simulink model "VSCHVDCunitblackstart"  (R2025b)
settings: Solver=VariableStepAuto  StartTime=0  StopTime=25  FixedStep=5e-5  RelTol=1e-3
PreLoadFcn:
  | HVDCParameters;
  | BlackStartMMCParameters;
undefined symbols (not defined in the file): DiscIntNeverNeededParam, FRated, frt, gGFM, grid, Lbase, Lr, Lt, lvrt, mGFM, mpptOmega, mpptWindSpeed, Nm, pmsm, PRated, Rc, rpir, Rr, Rt, time, Tpir, Ts, Vbase, Vdcs0, VRated, Vt2, windController, windTurbine, Zbase
libraries: fl_lib x47, ee_lib x41, nesl_utility x33, eeGeneralControl x13, eeTransforms x12, slpidlib x8, eeSinusoidalMeasurementV2 x4, simulink x2, eeSinusoidalMeasurement x1, eeStairGenerator x1
(part 4 of 5)

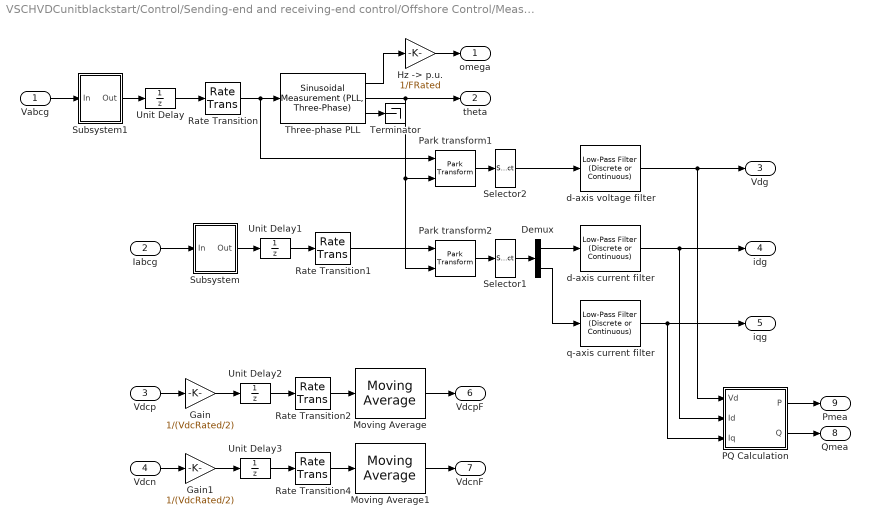
== system VSCHVDCunitblackstart/Control/Sending-end and receiving-end control/Offshore Control/Measurements ==
  Vabcg : Inport
  Iabcg : Inport  Port=2
  Vdcp : Inport  Port=3
  Vdcn : Inport  Port=4
  Demux : Demux  Outputs=2
  Gain : Gain  Gain=1/(VdcRated/2)
  Gain1 : Gain  Gain=1/(VdcRated/2)
  "Hz -> p.u." : Gain  Gain=1/FRated
  Moving Average : eeGeneralControl/Moving Average  VariantControl=Variant1  LabelModeActiveChoice=Discrete  f=FRated  x0=Vdcr0/2/(VdcRated/2)  BufferSize=8192  Ts=Tsc
  Moving Average1 : eeGeneralControl/Moving Average  VariantControl=Variant1  LabelModeActiveChoice=Discrete  f=FRated  x0=Vdcr0/2/(VdcRated/2)  BufferSize=8192  Ts=Tsc
  PQ Calculation : Subsystem
  Park transform1 : eeTransforms/Park Transform  AxisAlignment=Q-axis  PowerInvariant=off
  Park transform2 : eeTransforms/Park Transform  AxisAlignment=Q-axis  PowerInvariant=off
  Rate Transition : RateTransition  InitialCondition=Vabcgr0  OutPortSampleTime=Tsc
  Rate Transition1 : RateTransition  InitialCondition=Iabcgr0  OutPortSampleTime=Tsc
  Rate Transition2 : RateTransition  InitialCondition=Vdcr0/2/(VdcRated/2)  OutPortSampleTime=Tsc
  Rate Transition4 : RateTransition  InitialCondition=Vdcr0/2/(VdcRated/2)  OutPortSampleTime=Tsc
  Selector1 : Selector  InputPortWidth=3  IndexOptions=Index vector (dialog)  Indices=[1 2]  OutputSizes=1
  Selector2 : Selector  InputPortWidth=3  IndexOptions=Index vector (dialog)  Indices=[1]  OutputSizes=1
  Subsystem : Subsystem
  Subsystem1 : Subsystem
  Terminator : Terminator
  Three-phase PLL : eeSinusoidalMeasurement/Sinusoidal Measurement (PLL, Three-Phase)  Kp_LF=45  Ki_LF=1250  F0=FRated  Theta0=Vphaser0  Ts=Tsc
  Unit Delay : UnitDelay  InitialCondition=Vabcgr0  SampleTime=Ts  HasFrameUpgradeWarning=on
  Unit Delay1 : UnitDelay  InitialCondition=Iabcgr0  SampleTime=Ts  HasFrameUpgradeWarning=on
  Unit Delay2 : UnitDelay  InitialCondition=Vdcr0/2/(VdcRated/2)  SampleTime=Ts  HasFrameUpgradeWarning=on
  Unit Delay3 : UnitDelay  InitialCondition=Vdcr0/2/(VdcRated/2)  SampleTime=Ts  HasFrameUpgradeWarning=on
  d-axis current filter : eeGeneralControl/Low-Pass Filter (Discrete or Continuous)  K=1  T=5e-3  B=inf  A=-inf  init_option=Specify as parameter  x0=0  Ts=Tsc
  d-axis voltage filter : eeGeneralControl/Low-Pass Filter (Discrete or Continuous)  K=1  T=5e-3  B=inf  A=-inf  init_option=Specify as parameter  x0=0  Ts=Tsc
  q-axis current filter : eeGeneralControl/Low-Pass Filter (Discrete or Continuous)  K=1  T=5e-3  B=inf  A=-inf  init_option=Specify as parameter  x0=0  Ts=Tsc
  omega : Outport  VectorParamsAs1DForOutWhenUnconnected=off
  theta : Outport  Port=2  VectorParamsAs1DForOutWhenUnconnected=off
  Vdg : Outport  Port=3  VectorParamsAs1DForOutWhenUnconnected=off
  idg : Outport  Port=4  VectorParamsAs1DForOutWhenUnconnected=off
  iqg : Outport  Port=5  VectorParamsAs1DForOutWhenUnconnected=off
  VdcpF : Outport  Port=6  VectorParamsAs1DForOutWhenUnconnected=off
  VdcnF : Outport  Port=7  VectorParamsAs1DForOutWhenUnconnected=off
  Qmea : Outport  Port=8  VectorParamsAs1DForOutWhenUnconnected=off
  Pmea : Outport  Port=9  VectorParamsAs1DForOutWhenUnconnected=off
  wires:
  Moving Average1/1 -> VdcnF/1
  Vdcn/1 -> Gain1/1
  Rate Transition4/1 -> Moving Average1/1
  Gain1/1 -> Unit Delay3/1
  PQ Calculation/2(Q) -> Qmea/1
  PQ Calculation/1(P) -> Pmea/1
  Selector2/1 -> d-axis voltage filter/1
  d-axis current filter/1 -> idg/1, PQ Calculation/2(Id)
  Rate Transition1/1 -> Park transform2/1
  Rate Transition/1 -> Three-phase PLL/1, Park transform1/1
  d-axis voltage filter/1 -> PQ Calculation/1(Vd), Vdg/1
  Park transform2/1 -> Selector1/1
  Demux/1 -> d-axis current filter/1
  Gain/1 -> Unit Delay2/1
  Vdcp/1 -> Gain/1
  Demux/2 -> q-axis current filter/1
  Three-phase PLL/1 -> "Hz -> p.u."/1
  Park transform1/1 -> Selector2/1
  Three-phase PLL/2 -> Park transform1/2, Park transform2/2, theta/1
  Selector1/1 -> Demux/1
  Three-phase PLL/3 -> Terminator/1
  Moving Average/1 -> VdcpF/1
  "Hz -> p.u."/1 -> omega/1
  Iabcg/1 -> Subsystem/1(In)
  Vabcg/1 -> Subsystem1/1(In)
  Rate Transition2/1 -> Moving Average/1
  q-axis current filter/1 -> iqg/1, PQ Calculation/3(Iq)
  Unit Delay2/1 -> Rate Transition2/1
  Unit Delay3/1 -> Rate Transition4/1
  Unit Delay/1 -> Rate Transition/1
  Subsystem/1(Out) -> Unit Delay1/1
  Unit Delay1/1 -> Rate Transition1/1
  Subsystem1/1(Out) -> Unit Delay/1

== system VSCHVDCunitblackstart/Control/Sending-end and receiving-end control/Onshore Control/Control ==
  Vdref : Inport
  Vqref : Inport  Port=2
  Vdcp : Inport  Port=3
  Vdcn : Inport  Port=4
  Vdmea : Inport  Port=5
  Vqmea : Inport  Port=6
  theta : Inport  Port=7
  Active and reactive power control : Subsystem
  Add3 : Sum
  Constant : Constant  Value=0  SampleTime=Tsc
  Divide : Product  Inputs=*/
  Gain : Gain  Gain=2
  Gain5 : Gain  Gain=0.5*VdcRated/Vbase
  Inverse Park Transform : eeTransforms/Inverse Park Transform  AxisAlignment=Q-axis  PowerInvariant=off
  Mux1 : Mux  Inputs=3
  PWM generator : Subsystem
  S : Outport
  wires:
  Vdmea/1 -> Active and reactive power control/2(Vdmea)
  Vqmea/1 -> Active and reactive power control/4(Vqmea)
  PWM generator/1(S) -> S/1
  Vdref/1 -> Active and reactive power control/1(Vd)
  Vqref/1 -> Active and reactive power control/3(Vqref)
  Vdcn/1 -> Add3/2
  Vdcp/1 -> Add3/1
  Inverse Park Transform/1 -> Divide/1
  Gain5/1 -> Divide/2
  Add3/1 -> Gain5/1
  Divide/1 -> Gain/1
  Gain/1 -> PWM generator/1(Vref)
  Mux1/1 -> Inverse Park Transform/1
  theta/1 -> Inverse Park Transform/2
  Active and reactive power control/1(idRef) -> Mux1/1
  Constant/1 -> Mux1/3
  Active and reactive power control/2(iqRef) -> Mux1/2

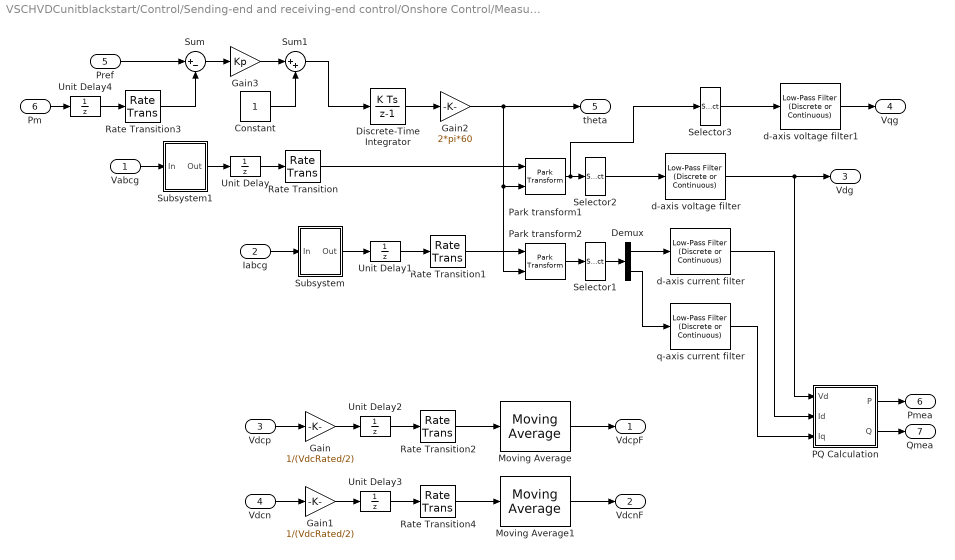
== system VSCHVDCunitblackstart/Control/Sending-end and receiving-end control/Onshore Control/Measurements ==
  Vabcg : Inport
  Iabcg : Inport  Port=2
  Vdcp : Inport  Port=3
  Vdcn : Inport  Port=4
  Pref : Inport  Port=5
  Pm : Inport  Port=6
  Constant : Constant
  Demux : Demux  Outputs=2
  Discrete-Time Integrator : DiscreteIntegrator  InitialCondition=1  SampleTime=-1  ICPrevOutput=DiscIntNeverNeededParam  ICPrevScaledInput=DiscIntNeverNeededParam
  Gain : Gain  Gain=1/(VdcRated/2)
  Gain1 : Gain  Gain=1/(VdcRated/2)
  Gain2 : Gain  Gain=2*pi*60
  Gain3 : Gain  Gain=Kp
  Moving Average : eeGeneralControl/Moving Average  VariantControl=Variant1  LabelModeActiveChoice=Discrete  f=FRated  x0=Vdcs0/2/(VdcRated/2)  BufferSize=8192  Ts=Tsc
  Moving Average1 : eeGeneralControl/Moving Average  VariantControl=Variant1  LabelModeActiveChoice=Discrete  f=FRated  x0=Vdcs0/2/(VdcRated/2)  BufferSize=8192  Ts=Tsc
  PQ Calculation : Subsystem
  Park transform1 : eeTransforms/Park Transform  AxisAlignment=Q-axis  PowerInvariant=off
  Park transform2 : eeTransforms/Park Transform  AxisAlignment=Q-axis  PowerInvariant=off
  Rate Transition : RateTransition  InitialCondition=Vabcgs0  OutPortSampleTime=Tsc
  Rate Transition1 : RateTransition  InitialCondition=Iabcgs0  OutPortSampleTime=Tsc
  Rate Transition2 : RateTransition  InitialCondition=Vdcs0/2/(VdcRated/2)  OutPortSampleTime=Tsc
  Rate Transition3 : RateTransition  InitialCondition=Vabcgs0  OutPortSampleTime=Tsc
  Rate Transition4 : RateTransition  InitialCondition=Vdcs0/2/(VdcRated/2)  OutPortSampleTime=Tsc
  Selector1 : Selector  InputPortWidth=3  IndexOptions=Index vector (dialog)  Indices=[1 2]  OutputSizes=1
  Selector2 : Selector  InputPortWidth=3  IndexOptions=Index vector (dialog)  Indices=[1]  OutputSizes=1
  Selector3 : Selector  InputPortWidth=3  IndexOptions=Index vector (dialog)  Indices=[2]  OutputSizes=1
  Subsystem : Subsystem
  Subsystem1 : Subsystem
  Sum : Sum  Inputs=|+-
  Sum1 : Sum  Inputs=|++
  Unit Delay : UnitDelay  InitialCondition=Vabcgs0  SampleTime=Ts  HasFrameUpgradeWarning=on
  Unit Delay1 : UnitDelay  InitialCondition=Iabcgs0  SampleTime=Ts  HasFrameUpgradeWarning=on
  Unit Delay2 : UnitDelay  InitialCondition=Vdcs0/2/(VdcRated/2)  SampleTime=Ts  HasFrameUpgradeWarning=on
  Unit Delay3 : UnitDelay  InitialCondition=Vdcs0/2/(VdcRated/2)  SampleTime=Ts  HasFrameUpgradeWarning=on
  Unit Delay4 : UnitDelay  InitialCondition=Vabcgs0  SampleTime=Ts  HasFrameUpgradeWarning=on
  d-axis current filter : eeGeneralControl/Low-Pass Filter (Discrete or Continuous)  K=1  T=5e-3  B=inf  A=-inf  init_option=Specify as parameter  x0=0  Ts=Tsc
  d-axis voltage filter : eeGeneralControl/Low-Pass Filter (Discrete or Continuous)  K=1  T=5e-3  B=inf  A=-inf  init_option=Specify as parameter  x0=0  Ts=Tsc
  d-axis voltage filter1 : eeGeneralControl/Low-Pass Filter (Discrete or Continuous)  K=1  T=5e-3  B=inf  A=-inf  init_option=Specify as parameter  x0=0  Ts=Tsc
  q-axis current filter : eeGeneralControl/Low-Pass Filter (Discrete or Continuous)  K=1  T=5e-3  B=inf  A=-inf  init_option=Specify as parameter  x0=0  Ts=Tsc
  VdcpF : Outport  VectorParamsAs1DForOutWhenUnconnected=off
  VdcnF : Outport  Port=2  VectorParamsAs1DForOutWhenUnconnected=off
  Vdg : Outport  Port=3  VectorParamsAs1DForOutWhenUnconnected=off
  Vqg : Outport  Port=4  VectorParamsAs1DForOutWhenUnconnected=off
  theta : Outport  Port=5  VectorParamsAs1DForOutWhenUnconnected=off
  Pmea : Outport  Port=6  VectorParamsAs1DForOutWhenUnconnected=off
  Qmea : Outport  Port=7  VectorParamsAs1DForOutWhenUnconnected=off
  wires:
  Rate Transition2/1 -> Moving Average/1
  Iabcg/1 -> Subsystem/1(In)
  Selector1/1 -> Demux/1
  Park transform1/1 -> Selector3/1, Selector2/1
  Demux/2 -> q-axis current filter/1
  Vdcp/1 -> Gain/1
  Demux/1 -> d-axis current filter/1
  Park transform2/1 -> Selector1/1
  d-axis voltage filter/1 -> Vdg/1, PQ Calculation/1(Vd)
  Rate Transition/1 -> Park transform1/1
  Rate Transition1/1 -> Park transform2/1
  Selector2/1 -> d-axis voltage filter/1
  PQ Calculation/1(P) -> Pmea/1
  PQ Calculation/2(Q) -> Qmea/1
  Rate Transition4/1 -> Moving Average1/1
  Vdcn/1 -> Gain1/1
  Discrete-Time Integrator/1 -> Gain2/1
  Unit Delay/1 -> Rate Transition/1
  Unit Delay2/1 -> Rate Transition2/1
  Unit Delay3/1 -> Rate Transition4/1
  Gain/1 -> Unit Delay2/1
  Gain1/1 -> Unit Delay3/1
  Vabcg/1 -> Subsystem1/1(In)
  Subsystem/1(Out) -> Unit Delay1/1
  d-axis current filter/1 -> PQ Calculation/2(Id)
  q-axis current filter/1 -> PQ Calculation/3(Iq)
  Moving Average/1 -> VdcpF/1
  Moving Average1/1 -> VdcnF/1
  Unit Delay1/1 -> Rate Transition1/1
  Subsystem1/1(Out) -> Unit Delay/1
  Gain2/1 -> Park transform2/2, Park transform1/2, theta/1
  Pref/1 -> Sum/1
  Pm/1 -> Unit Delay4/1
  Sum/1 -> Gain3/1
  Gain3/1 -> Sum1/1
  Sum1/1 -> Discrete-Time Integrator/1
  Constant/1 -> Sum1/2
  Rate Transition3/1 -> Sum/2
  Unit Delay4/1 -> Rate Transition3/1
  Selector3/1 -> d-axis voltage filter1/1
  d-axis voltage filter1/1 -> Vqg/1

== system VSCHVDCunitblackstart/Wind Farm/Wind Farm/CB1/Subsystem1 ==
  input0 : Inport
  Gain : Gain  Gain=1e9
  Phase Splitter : ee_lib/Connectors & References/Phase Splitter
  Phase Splitter1 : ee_lib/Connectors & References/Phase Splitter
  Simulink-PS Converter : nesl_utility/Simulink-PS Converter  PhysicalDomain=network_engine_domain  SubClassName=ps_input  LeftPortType=input  RightPortType=output  PseudoPeriodic=off  Frequencies=[]  NoiseDistribution=none  NoiseParameters=[]  Unit=1  AffineConversion=off  FilteringAndDerivatives=provide  SimscapeFilterOrder=1  InputFilterTimeConstant=0.001  UdotUserProvided=0
  Variable Resistor : fl_lib/Electrical/Electrical Elements/Variable Resistor  Rmin=1e-4 Ohm  thermalEnable=false  thermal_mass=1 J/K  i_specify=off  i_priority=None  i=0 A  i_nominal_specify=off  i_nominal_value=1  i_nominal_unit=A  v_specify=off  v_priority=None  v=0 V  v_nominal_specify=off  v_nominal_value=1  v_nominal_unit=V  T_specify=off  T_priority=None  T=300 K  T_nominal_specify=off  T_nominal_value=1  T_nominal_unit=K
  Variable Resistor1 : fl_lib/Electrical/Electrical Elements/Variable Resistor  Rmin=1e-4 Ohm  thermalEnable=false  thermal_mass=1 J/K  i_specify=off  i_priority=None  i=0 A  i_nominal_specify=off  i_nominal_value=1  i_nominal_unit=A  v_specify=off  v_priority=None  v=0 V  v_nominal_specify=off  v_nominal_value=1  v_nominal_unit=V  T_specify=off  T_priority=None  T=300 K  T_nominal_specify=off  T_nominal_value=1  T_nominal_unit=K
  Variable Resistor2 : fl_lib/Electrical/Electrical Elements/Variable Resistor  Rmin=1e-4 Ohm  thermalEnable=false  thermal_mass=1 J/K  i_specify=off  i_priority=None  i=0 A  i_nominal_specify=off  i_nominal_value=1  i_nominal_unit=A  v_specify=off  v_priority=None  v=0 V  v_nominal_specify=off  v_nominal_value=1  v_nominal_unit=V  T_specify=off  T_priority=None  T=300 K  T_nominal_specify=off  T_nominal_value=1  T_nominal_unit=K
  Conn1 : PMIOPort  Side=Left
  Conn2 : PMIOPort  Port=2  Side=Right
  wires:
  input0/1 -> Gain/1
  Gain/1 -> Simulink-PS Converter/1
  connections:
  Simulink-PS Converter/RConn1 -- Variable Resistor2/LConn1 -- Variable Resistor1/LConn1 -- Variable Resistor/LConn1
  Phase Splitter/LConn1 -- Conn2/RConn1
  Phase Splitter/RConn1 -- Variable Resistor/LConn2
  Phase Splitter/RConn2 -- Variable Resistor1/LConn2
  Phase Splitter/RConn3 -- Variable Resistor2/LConn2
  Phase Splitter1/LConn1 -- Conn1/RConn1
  Variable Resistor/RConn1 -- Phase Splitter1/RConn1
  Phase Splitter1/RConn2 -- Variable Resistor1/RConn1
  Variable Resistor2/RConn1 -- Phase Splitter1/RConn3

== system VSCHVDCunitblackstart/Wind Farm/Wind Farm/PLL & Measurements/Measurement1 ==
  u : Inport
  Ig : Outport
  wires:
  u/1 -> Ig/1

== system VSCHVDCunitblackstart/Wind Farm/Wind Farm/PLL & Measurements/Measurement2 ==
  u : Inport
  Vg : Outport
  wires:
  u/1 -> Vg/1

== system VSCHVDCunitblackstart/Wind Farm/Wind Farm/PLL & Measurements/PLL ==
  abc : Inport
  Ig : Inport  Port=2
  Demux : Demux  Outputs=3
  Demux1 : Demux  Outputs=3
  Park Transform : eeTransforms/Park Transform  AxisAlignment=Q-axis  PowerInvariant=off
  Park Transform1 : eeTransforms/Park Transform  AxisAlignment=Q-axis  PowerInvariant=off
  "Sinusoidal Measurement (PLL, Three-Phase)1" : eeSinusoidalMeasurementV2/Sinusoidal Measurement (PLL, Three-Phase)  InputFilter=on  InputNormalization=off  Kp_LF=pll.kp  Ki_LF=pll.ki  F0=grid.frequency  Theta0=0  Ts=Ts
      settings: LibrarySourceBlock=|
      | ee_sl_lib/Measurements/Sinusoidal Measurement
      | (PLL, Three-Phase)
  Terminator : Terminator
  Terminator1 : Terminator
  abc1 : InportShadow
  mag : Outport
  freq : Outport  Port=2
  angle : Outport  Port=3
  Vd : Outport  Port=4
  Vq : Outport  Port=5
  Id : Outport  Port=6
  Iq : Outport  Port=7
  wires:
  Demux/3 -> Terminator/1
  Park Transform/1 -> Demux/1
  Demux/1 -> Vd/1
  Demux/2 -> Vq/1
  "Sinusoidal Measurement (PLL, Three-Phase)1"/3 -> mag/1
  "Sinusoidal Measurement (PLL, Three-Phase)1"/2 -> angle/1, Park Transform/2, Park Transform1/2
  Ig/1 -> Park Transform1/1
  Demux1/2 -> Iq/1
  Park Transform1/1 -> Demux1/1
  Demux1/1 -> Id/1
  Demux1/3 -> Terminator1/1
  abc1/1 -> Park Transform/1
  abc/1 -> "Sinusoidal Measurement (PLL, Three-Phase)1"/1
  "Sinusoidal Measurement (PLL, Three-Phase)1"/1 -> freq/1

== system VSCHVDCunitblackstart/Wind Farm/Wind Farm/Voltage VAR Control & LVRT, FRT/Frequency RideThrough ==
  f : Inport
  Avoid Operation : Subsystem
  Discrete-Time Integrator1 : DiscreteIntegrator  ExternalReset=either  SampleTime=Ts  ICPrevOutput=DiscIntNeverNeededParam  ICPrevScaledInput=DiscIntNeverNeededParam
  Duration of f<fth : Lookup_n-D  NumberOfTableDimensions=1  BreakpointsForDimension1=(1+[-0.021,-0.02,0.02,0.021])*grid.frequency  Table=[1,0,0,1]  InterpMethod=Flat  InternalRulePriority=Speed  RndMeth=Simplest
  Frequency vs Trip time : Lookup_n-D  NumberOfTableDimensions=1  BreakpointsForDimension1=frt.frequency  Table=frt.time  InterpMethod=Flat  InternalRulePriority=Speed  RndMeth=Simplest
  GreaterThan : RelationalOperator  Operator=>  OutDataTypeStr=boolean  RndMeth=Simplest  InputSameDT=off
  Trip  Signal : Outport
  wires:
  Discrete-Time Integrator1/1 -> GreaterThan/1
  Frequency vs Trip time/1 -> GreaterThan/2
  GreaterThan/1 -> Trip  Signal/1
  Duration of f<fth/1 -> Discrete-Time Integrator1/2, Discrete-Time Integrator1/1
  Avoid Operation/1(f) -> Duration of f<fth/1, Frequency vs Trip time/1
  f/1 -> Avoid Operation/1(f_in)

== system VSCHVDCunitblackstart/Wind Farm/Wind Farm/Voltage VAR Control & LVRT, FRT/LVRT Characterstics ==
  Vmag : Inport
  Discrete-Time Integrator1 : DiscreteIntegrator  ExternalReset=either  SampleTime=Ts  ICPrevOutput=DiscIntNeverNeededParam  ICPrevScaledInput=DiscIntNeverNeededParam
  Duration of Vmag<Vth : Lookup_n-D  NumberOfTableDimensions=1  BreakpointsForDimension1=[0,.9,0.91,1.2]  Table=[1,1,0,0]  InterpMethod=Flat  InternalRulePriority=Speed  RndMeth=Simplest
  Gain1 : Gain  Gain=-1
  GreaterThan : RelationalOperator  Operator=>  OutDataTypeStr=boolean  RndMeth=Simplest  InputSameDT=off
  Saturation2 : Saturate  UpperLimit=1/8  LowerLimit=-1
  Vmag vs Trip time : Lookup_n-D  NumberOfTableDimensions=1  BreakpointsForDimension1=lvrt.voltage  Table=lvrt.time  InterpMethod=Flat  InternalRulePriority=Speed  RndMeth=Simplest
  Vmag vs iq : Lookup_n-D  NumberOfTableDimensions=1  BreakpointsForDimension1=lvrt.voltageiq  Table=lvrt.iq  InternalRulePriority=Speed  RndMeth=Simplest
  Trip Signal : Outport
  iq : Outport  Port=2
  wires:
  Duration of Vmag<Vth/1 -> Discrete-Time Integrator1/2, Discrete-Time Integrator1/1
  GreaterThan/1 -> Trip Signal/1
  Discrete-Time Integrator1/1 -> GreaterThan/1
  Vmag vs Trip time/1 -> GreaterThan/2
  Vmag vs iq/1 -> Saturation2/1
  Gain1/1 -> iq/1
  Saturation2/1 -> Gain1/1
  Vmag/1 -> Vmag vs iq/1, Vmag vs Trip time/1, Duration of Vmag<Vth/1

== system VSCHVDCunitblackstart/Wind Farm/Wind Farm/Voltage VAR Control & LVRT, FRT/Voltage Control ==
  In1 : Inport
  In2 : Inport  Port=2
  Constant2 : Constant  Value=0
  Gain : Gain  Gain=windController.mv
  Sum2 : Sum  Inputs=|+-
  Switch1 : Switch  Threshold=.9  SaturateOnIntegerOverflow=off  InputSameDT=off
  Out1 : Outport
  wires:
  Gain/1 -> Out1/1
  Sum2/1 -> Switch1/1
  Switch1/1 -> Gain/1
  In1/1 -> Sum2/2, Switch1/2
  Constant2/1 -> Switch1/3
  In2/1 -> Sum2/1

== system VSCHVDCunitblackstart/Wind Farm/Wind Farm1/CB1/Subsystem1 ==
  input0 : Inport
  Gain : Gain  Gain=1e9
  Phase Splitter : ee_lib/Connectors & References/Phase Splitter
  Phase Splitter1 : ee_lib/Connectors & References/Phase Splitter
  Simulink-PS Converter : nesl_utility/Simulink-PS Converter  PhysicalDomain=network_engine_domain  SubClassName=ps_input  LeftPortType=input  RightPortType=output  PseudoPeriodic=off  Frequencies=[]  NoiseDistribution=none  NoiseParameters=[]  Unit=1  AffineConversion=off  FilteringAndDerivatives=provide  SimscapeFilterOrder=1  InputFilterTimeConstant=0.001  UdotUserProvided=0
  Variable Resistor : fl_lib/Electrical/Electrical Elements/Variable Resistor  Rmin=1e-4 Ohm  thermalEnable=false  thermal_mass=1 J/K  i_specify=off  i_priority=None  i=0 A  i_nominal_specify=off  i_nominal_value=1  i_nominal_unit=A  v_specify=off  v_priority=None  v=0 V  v_nominal_specify=off  v_nominal_value=1  v_nominal_unit=V  T_specify=off  T_priority=None  T=300 K  T_nominal_specify=off  T_nominal_value=1  T_nominal_unit=K
  Variable Resistor1 : fl_lib/Electrical/Electrical Elements/Variable Resistor  Rmin=1e-4 Ohm  thermalEnable=false  thermal_mass=1 J/K  i_specify=off  i_priority=None  i=0 A  i_nominal_specify=off  i_nominal_value=1  i_nominal_unit=A  v_specify=off  v_priority=None  v=0 V  v_nominal_specify=off  v_nominal_value=1  v_nominal_unit=V  T_specify=off  T_priority=None  T=300 K  T_nominal_specify=off  T_nominal_value=1  T_nominal_unit=K
  Variable Resistor2 : fl_lib/Electrical/Electrical Elements/Variable Resistor  Rmin=1e-4 Ohm  thermalEnable=false  thermal_mass=1 J/K  i_specify=off  i_priority=None  i=0 A  i_nominal_specify=off  i_nominal_value=1  i_nominal_unit=A  v_specify=off  v_priority=None  v=0 V  v_nominal_specify=off  v_nominal_value=1  v_nominal_unit=V  T_specify=off  T_priority=None  T=300 K  T_nominal_specify=off  T_nominal_value=1  T_nominal_unit=K
  Conn1 : PMIOPort  Side=Left
  Conn2 : PMIOPort  Port=2  Side=Right
  wires:
  input0/1 -> Gain/1
  Gain/1 -> Simulink-PS Converter/1
  connections:
  Simulink-PS Converter/RConn1 -- Variable Resistor2/LConn1 -- Variable Resistor1/LConn1 -- Variable Resistor/LConn1
  Phase Splitter/LConn1 -- Conn2/RConn1
  Phase Splitter/RConn1 -- Variable Resistor/LConn2
  Phase Splitter/RConn2 -- Variable Resistor1/LConn2
  Phase Splitter/RConn3 -- Variable Resistor2/LConn2
  Phase Splitter1/LConn1 -- Conn1/RConn1
  Variable Resistor/RConn1 -- Phase Splitter1/RConn1
  Phase Splitter1/RConn2 -- Variable Resistor1/RConn1
  Variable Resistor2/RConn1 -- Phase Splitter1/RConn3

== system VSCHVDCunitblackstart/Wind Farm/Wind Farm1/PLL & Measurements/Measurement1 ==
  u : Inport
  Ig : Outport
  wires:
  u/1 -> Ig/1

== system VSCHVDCunitblackstart/Wind Farm/Wind Farm1/PLL & Measurements/Measurement2 ==
  u : Inport
  Vg : Outport
  wires:
  u/1 -> Vg/1

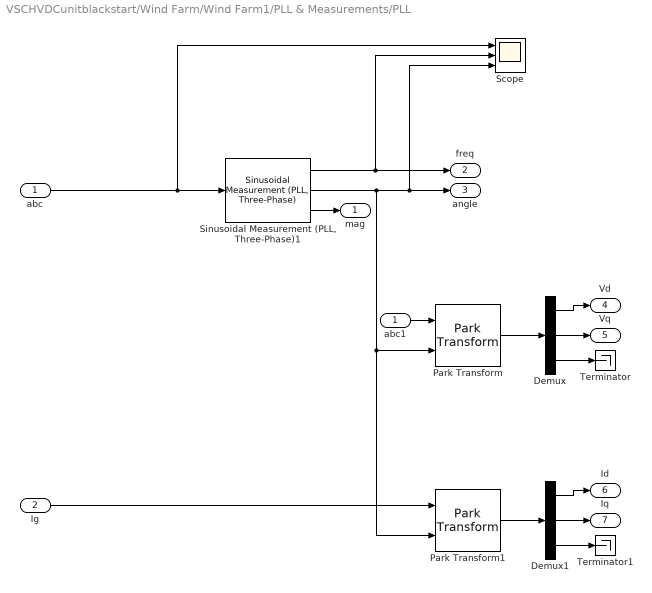
== system VSCHVDCunitblackstart/Wind Farm/Wind Farm1/PLL & Measurements/PLL ==
  abc : Inport
  Ig : Inport  Port=2
  Demux : Demux  Outputs=3
  Demux1 : Demux  Outputs=3
  Park Transform : eeTransforms/Park Transform  AxisAlignment=Q-axis  PowerInvariant=off
  Park Transform1 : eeTransforms/Park Transform  AxisAlignment=Q-axis  PowerInvariant=off
  Scope : Scope  NumInputPorts=3
      settings: ActiveDisplayYMinimum=-1.5640635972149539  ActiveDisplayYMaximum=1.5640663714492395  DataLoggingVariableName=ScopeData5
  "Sinusoidal Measurement (PLL, Three-Phase)1" : eeSinusoidalMeasurementV2/Sinusoidal Measurement (PLL, Three-Phase)  InputFilter=on  InputNormalization=off  Kp_LF=pll.kp  Ki_LF=pll.ki  F0=grid.frequency  Theta0=0  Ts=Ts
      settings: LibrarySourceBlock=|
      | ee_sl_lib/Measurements/Sinusoidal Measurement
      | (PLL, Three-Phase)
  Terminator : Terminator
  Terminator1 : Terminator
  abc1 : InportShadow
  mag : Outport
  freq : Outport  Port=2
  angle : Outport  Port=3
  Vd : Outport  Port=4
  Vq : Outport  Port=5
  Id : Outport  Port=6
  Iq : Outport  Port=7
  wires:
  Demux/3 -> Terminator/1
  Park Transform/1 -> Demux/1
  Demux/1 -> Vd/1
  Demux/2 -> Vq/1
  "Sinusoidal Measurement (PLL, Three-Phase)1"/3 -> mag/1
  "Sinusoidal Measurement (PLL, Three-Phase)1"/2 -> Scope/3, angle/1, Park Transform/2, Park Transform1/2
  Ig/1 -> Park Transform1/1
  Demux1/2 -> Iq/1
  Park Transform1/1 -> Demux1/1
  Demux1/1 -> Id/1
  Demux1/3 -> Terminator1/1
  abc1/1 -> Park Transform/1
  abc/1 -> Scope/1, "Sinusoidal Measurement (PLL, Three-Phase)1"/1
  "Sinusoidal Measurement (PLL, Three-Phase)1"/1 -> Scope/2, freq/1

== system VSCHVDCunitblackstart/Wind Farm/Wind Farm1/Voltage VAR Control & LVRT, FRT/Frequency RideThrough ==
  f : Inport
  Avoid Operation : Subsystem
  Discrete-Time Integrator1 : DiscreteIntegrator  ExternalReset=either  SampleTime=Ts  ICPrevOutput=DiscIntNeverNeededParam  ICPrevScaledInput=DiscIntNeverNeededParam
  Duration of f<fth : Lookup_n-D  NumberOfTableDimensions=1  BreakpointsForDimension1=(1+[-0.021,-0.02,0.02,0.021])*grid.frequency  Table=[1,0,0,1]  InterpMethod=Flat  InternalRulePriority=Speed  RndMeth=Simplest
  Frequency vs Trip time : Lookup_n-D  NumberOfTableDimensions=1  BreakpointsForDimension1=frt.frequency  Table=frt.time  InterpMethod=Flat  InternalRulePriority=Speed  RndMeth=Simplest
  GreaterThan : RelationalOperator  Operator=>  OutDataTypeStr=boolean  RndMeth=Simplest  InputSameDT=off
  Trip  Signal : Outport
  wires:
  Discrete-Time Integrator1/1 -> GreaterThan/1
  Frequency vs Trip time/1 -> GreaterThan/2
  GreaterThan/1 -> Trip  Signal/1
  Duration of f<fth/1 -> Discrete-Time Integrator1/2, Discrete-Time Integrator1/1
  Avoid Operation/1(f) -> Duration of f<fth/1, Frequency vs Trip time/1
  f/1 -> Avoid Operation/1(f_in)

== system VSCHVDCunitblackstart/Wind Farm/Wind Farm1/Voltage VAR Control & LVRT, FRT/LVRT Characterstics ==
  Vmag : Inport
  Discrete-Time Integrator1 : DiscreteIntegrator  ExternalReset=either  SampleTime=Ts  ICPrevOutput=DiscIntNeverNeededParam  ICPrevScaledInput=DiscIntNeverNeededParam
  Duration of Vmag<Vth : Lookup_n-D  NumberOfTableDimensions=1  BreakpointsForDimension1=[0,.9,0.91,1.2]  Table=[1,1,0,0]  InterpMethod=Flat  InternalRulePriority=Speed  RndMeth=Simplest
  Gain1 : Gain  Gain=-1
  GreaterThan : RelationalOperator  Operator=>  OutDataTypeStr=boolean  RndMeth=Simplest  InputSameDT=off
  Saturation2 : Saturate  UpperLimit=1/8  LowerLimit=-1
  Vmag vs Trip time : Lookup_n-D  NumberOfTableDimensions=1  BreakpointsForDimension1=lvrt.voltage  Table=lvrt.time  InterpMethod=Flat  InternalRulePriority=Speed  RndMeth=Simplest
  Vmag vs iq : Lookup_n-D  NumberOfTableDimensions=1  BreakpointsForDimension1=lvrt.voltageiq  Table=lvrt.iq  InternalRulePriority=Speed  RndMeth=Simplest
  Trip Signal : Outport
  iq : Outport  Port=2
  wires:
  Duration of Vmag<Vth/1 -> Discrete-Time Integrator1/2, Discrete-Time Integrator1/1
  GreaterThan/1 -> Trip Signal/1
  Discrete-Time Integrator1/1 -> GreaterThan/1
  Vmag vs Trip time/1 -> GreaterThan/2
  Vmag vs iq/1 -> Saturation2/1
  Gain1/1 -> iq/1
  Saturation2/1 -> Gain1/1
  Vmag/1 -> Vmag vs iq/1, Vmag vs Trip time/1, Duration of Vmag<Vth/1

== system VSCHVDCunitblackstart/Wind Farm/Wind Farm1/Voltage VAR Control & LVRT, FRT/Voltage Control ==
  In1 : Inport
  In2 : Inport  Port=2
  Constant2 : Constant  Value=0
  Gain : Gain  Gain=windController.mv
  Sum2 : Sum  Inputs=|+-
  Switch1 : Switch  Threshold=.9  SaturateOnIntegerOverflow=off  InputSameDT=off
  Out1 : Outport
  wires:
  Gain/1 -> Out1/1
  Sum2/1 -> Switch1/1
  Switch1/1 -> Gain/1
  In1/1 -> Sum2/2, Switch1/2
  Constant2/1 -> Switch1/3
  In2/1 -> Sum2/1

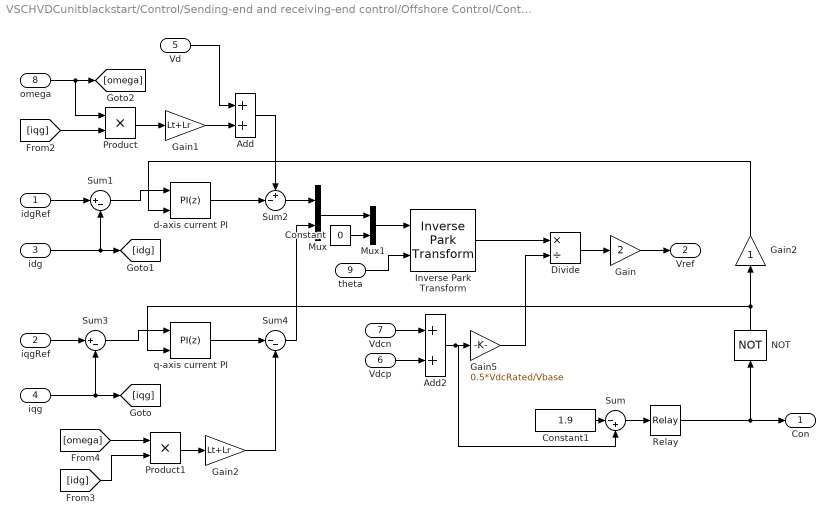
== system VSCHVDCunitblackstart/Control/Sending-end and receiving-end control/Offshore Control/Control/Current control ==
  idgRef : Inport
  iqgRef : Inport  Port=2
  idg : Inport  Port=3
  iqg : Inport  Port=4
  Vd : Inport  Port=5
  Vdcp : Inport  Port=6
  Vdcn : Inport  Port=7
  omega : Inport  Port=8
  theta : Inport  Port=9
  Add : Sum
  Add2 : Sum
  Constant : Constant  Value=0  SampleTime=Tsc
  Constant1 : Constant  Value=1.9  SampleTime=-1
  Divide : Product  Inputs=*/
  Gain : Gain  Gain=2
  Gain1 : Gain  Gain=Lt+Lr
  Gain2 : Gain
  "Gain2 " : Gain  Gain=Lt+Lr
  Gain5 : Gain  Gain=0.5*VdcRated/Vbase
  Inverse Park Transform : eeTransforms/Inverse Park Transform  AxisAlignment=Q-axis  PowerInvariant=off
  Mux : Mux  Inputs=2
  Mux1 : Mux  Inputs=2
  NOT : Logic  Operator=NOT  IconShape=distinctive  AllPortsSameDT=off  OutDataTypeStr=boolean
  Product : Product  Inputs=**
  Product1 : Product  Inputs=**
  Relay : Relay  OnSwitchValue=-0.01  OffSwitchValue=-0.5  OnOutputValue=0  OffOutputValue=1
  Sum : Sum  Inputs=|-+
  Sum1 : Sum  Inputs=|+-
  Sum2 : Sum  Inputs=+-|
  Sum3 : Sum  Inputs=|+-
  Sum4 : Sum  Inputs=|--
  d-axis current PI : slpidlib/PID Controller  Controller=PI  Form=Parallel  TimeDomain=Discrete-time  UseExternalTs=off  SampleTime=Tsc  IntegratorMethod=Forward Euler  FilterMethod=Forward Euler  ControllerParametersSource=internal  P=REnd_Id_PI(1)  I=REnd_Id_PI(2)  UseKiTs=off  D=0  UseExternalDerivativeSource=off  N=100  UseFilter=on  TunerSelectOption=Transfer Function Based (PID Tuner App)  InitialConditionSource=internal  InitialConditionForIntegrator=0  InitialConditionForFilter=0  DifferentiatorICPrevScaledInput=0  ExternalReset=rising  TrackingMode=off  Kt=1  LimitOutput=on  SatLimitsSource=internal  UpperSaturationLimit=(Rt+Rr)*40  LowerSaturationLimit=-(Rt+Rr)*40  LinearizeAsGain=on  AntiWindupMode=back-calculation  Kb=1000  LimitIntegrator=off  UpperIntegratorSaturationLimit=inf  LowerIntegratorSaturationLimit=-inf  POutMin=[]  POutMax=[]  IOutMin=[]  IOutMax=[]  DOutMin=[]  DOutMax=[]  NOutMin=[]  NOutMax=[]  SumOutMin=[]  SumOutMax=[]  SaturationOutMin=[]  SaturationOutMax=[]  PParamMin=[]  PParamMax=[]  IParamMin=[]  IParamMax=[]  DParamMin=[]  DParamMax=[]  NParamMin=[]  NParamMax=[]  KbParamMin=[]  KbParamMax=[]  KtParamMin=[]  KtParamMax=[]  KbOutMin=[]  KbOutMax=[]  KtOutMin=[]  KtOutMax=[]  IntegratorOutMin=[]  IntegratorOutMax=[]  FilterOutMin=[]  FilterOutMax=[]  SumI1OutMin=[]  SumI1OutMax=[]  SumI2OutMin=[]  SumI2OutMax=[]  SumI3OutMin=[]  SumI3OutMax=[]  SumI4OutMin=[]  SumI4OutMax=[]  SumDOutMin=[]  SumDOutMax=[]  DifferentiatorOutMin=[]  DifferentiatorOutMax=[]  FilterDiffOutCoefMin=[]  FilterDiffOutCoefMax=[]  ReciprocalOutMin=[]  ReciprocalOutMax=[]  SumDenOutMin=[]  SumDenOutMax=[]  SumNumOutMin=[]  SumNumOutMax=[]  DivideOutMin=[]  DivideOutMax=[]  UdiffTsProdOutMin=[]  UdiffTsProdOutMax=[]  NTsProdOutMin=[]  NTsProdOutMax=[]  UintegralTsProdOutMin=[]  UintegralTsProdOutMax=[]  UngainTsProdOutMin=[]  UngainTsProdOutMax=[]  ClampingZeroOutDataTypeStr=Inherit: Inherit via back propagation  ClampingZeroOutMin=[]  ClampingZeroOutMax=[]  FilterDenConstantOutDataTypeStr=Inherit: Inherit via back propagation  FilterDenConstantOutMin=[]  FilterDenConstantOutMax=[]  PCopyOutDataTypeStr=Inherit: Inherit via back propagation  PCopyOutMin=[]  PCopyOutMax=[]  NCopyOutDataTypeStr=Inherit: Inherit via back propagation  NCopyOutMin=[]  NCopyOutMax=[]  IntegratorContinuousStateAttributes=''  IntegratorStateMustResolveToSignalObject=off  IntegratorRTWStateStorageClass=Auto  FilterContinuousStateAttributes=''  FilterStateMustResolveToSignalObject=off  FilterRTWStateStorageClass=Auto  ParallelPVariant=InternalParameters  IdealPVariant=Disabled  IVariant=InternalParameters  DVariant=Disabled  IntegratorVariant=Discrete  SatVariant=Enabled  AWVariant=BackCalculation  PCopyVariant=Disabled  TRVariant=Disabled  FdbkBlocksVariant=Forward  IdealPFdbkVariant=Disabled  SatFdbkVariant=Disabled  DerivativeFilterVariant=Disabled  NVariant=Disabled  NCopyVariant=Disabled_SignalSpec  FilterICVariant=Disabled  IntegratorICVariant=InternalICs  ExternalResetVariant=ExternalReset  TRSumVariant=Passthrough  SumFdbkVariant=Disabled  SumVariant=Sum_PI  TsampFilterVariant=InternalTs  TsampNgainVariant=Passthrough  TsampIntegralVariant=Disabled_SignalSpec  ExternalSaturationOutDataTypeStr=Inherit: Same as second input  DerivativeSourceVariant=Disabled  PreIntVariant=InternalPreInt
  q-axis current PI : slpidlib/PID Controller  Controller=PI  Form=Parallel  TimeDomain=Discrete-time  UseExternalTs=off  SampleTime=Tsc  IntegratorMethod=Forward Euler  FilterMethod=Forward Euler  ControllerParametersSource=internal  P=REnd_Iq_PI(1)  I=REnd_Iq_PI(2)  UseKiTs=off  D=0  UseExternalDerivativeSource=off  N=100  UseFilter=on  TunerSelectOption=Transfer Function Based (PID Tuner App)  InitialConditionSource=internal  InitialConditionForIntegrator=0  InitialConditionForFilter=0  DifferentiatorICPrevScaledInput=0  ExternalReset=rising  TrackingMode=off  Kt=1  LimitOutput=on  SatLimitsSource=internal  UpperSaturationLimit=(Rt+Rr)*40  LowerSaturationLimit=-(Rt+Rr)*40  LinearizeAsGain=on  AntiWindupMode=back-calculation  Kb=1000  LimitIntegrator=off  UpperIntegratorSaturationLimit=inf  LowerIntegratorSaturationLimit=-inf  POutMin=[]  POutMax=[]  IOutMin=[]  IOutMax=[]  DOutMin=[]  DOutMax=[]  NOutMin=[]  NOutMax=[]  SumOutMin=[]  SumOutMax=[]  SaturationOutMin=[]  SaturationOutMax=[]  PParamMin=[]  PParamMax=[]  IParamMin=[]  IParamMax=[]  DParamMin=[]  DParamMax=[]  NParamMin=[]  NParamMax=[]  KbParamMin=[]  KbParamMax=[]  KtParamMin=[]  KtParamMax=[]  KbOutMin=[]  KbOutMax=[]  KtOutMin=[]  KtOutMax=[]  IntegratorOutMin=[]  IntegratorOutMax=[]  FilterOutMin=[]  FilterOutMax=[]  SumI1OutMin=[]  SumI1OutMax=[]  SumI2OutMin=[]  SumI2OutMax=[]  SumI3OutMin=[]  SumI3OutMax=[]  SumI4OutMin=[]  SumI4OutMax=[]  SumDOutMin=[]  SumDOutMax=[]  DifferentiatorOutMin=[]  DifferentiatorOutMax=[]  FilterDiffOutCoefMin=[]  FilterDiffOutCoefMax=[]  ReciprocalOutMin=[]  ReciprocalOutMax=[]  SumDenOutMin=[]  SumDenOutMax=[]  SumNumOutMin=[]  SumNumOutMax=[]  DivideOutMin=[]  DivideOutMax=[]  UdiffTsProdOutMin=[]  UdiffTsProdOutMax=[]  NTsProdOutMin=[]  NTsProdOutMax=[]  UintegralTsProdOutMin=[]  UintegralTsProdOutMax=[]  UngainTsProdOutMin=[]  UngainTsProdOutMax=[]  ClampingZeroOutDataTypeStr=Inherit: Inherit via back propagation  ClampingZeroOutMin=[]  ClampingZeroOutMax=[]  FilterDenConstantOutDataTypeStr=Inherit: Inherit via back propagation  FilterDenConstantOutMin=[]  FilterDenConstantOutMax=[]  PCopyOutDataTypeStr=Inherit: Inherit via back propagation  PCopyOutMin=[]  PCopyOutMax=[]  NCopyOutDataTypeStr=Inherit: Inherit via back propagation  NCopyOutMin=[]  NCopyOutMax=[]  IntegratorContinuousStateAttributes=''  IntegratorStateMustResolveToSignalObject=off  IntegratorRTWStateStorageClass=Auto  FilterContinuousStateAttributes=''  FilterStateMustResolveToSignalObject=off  FilterRTWStateStorageClass=Auto  ParallelPVariant=InternalParameters  IdealPVariant=Disabled  IVariant=InternalParameters  DVariant=Disabled  IntegratorVariant=Discrete  SatVariant=Enabled  AWVariant=BackCalculation  PCopyVariant=Disabled  TRVariant=Disabled  FdbkBlocksVariant=Forward  IdealPFdbkVariant=Disabled  SatFdbkVariant=Disabled  DerivativeFilterVariant=Disabled  NVariant=Disabled  NCopyVariant=Disabled_SignalSpec  FilterICVariant=Disabled  IntegratorICVariant=InternalICs  ExternalResetVariant=ExternalReset  TRSumVariant=Passthrough  SumFdbkVariant=Disabled  SumVariant=Sum_PI  TsampFilterVariant=InternalTs  TsampNgainVariant=Passthrough  TsampIntegralVariant=Disabled_SignalSpec  ExternalSaturationOutDataTypeStr=Inherit: Same as second input  DerivativeSourceVariant=Disabled  PreIntVariant=InternalPreInt
  Con : Outport
  Vref : Outport  Port=2
  wires:
  Mux/1 -> Mux1/1
  "Gain2 "/1 -> Sum4/2
  Vdcn/1 -> Add2/1
  Vdcp/1 -> Add2/2
  Gain5/1 -> Divide/2
  Sum3/1 -> q-axis current PI/1
  q-axis current PI/1 -> Sum4/1
  Sum1/1 -> d-axis current PI/1
  d-axis current PI/1 -> Sum2/2
  iqg/1 -> Sum3/2, [iqg]
  Divide/1 -> Gain/1
  Gain/1 -> Vref/1
  Sum2/1 -> Mux/1
  Gain1/1 -> Add/2
  theta/1 -> Inverse Park Transform/2
  idg/1 -> [idg], Sum1/2
  Add/1 -> Sum2/1
  Product1/1 -> "Gain2 "/1
  Sum4/1 -> Mux/2
  Product/1 -> Gain1/1
  [omega] -> Product1/1
  omega/1 -> [omega], Product/1
  [iqg] -> Product/2
  Mux1/1 -> Inverse Park Transform/1
  Inverse Park Transform/1 -> Divide/1
  Constant/1 -> Mux1/2
  [idg] -> Product1/2
  idgRef/1 -> Sum1/1
  Vd/1 -> Add/1
  iqgRef/1 -> Sum3/1
  Sum/1 -> Relay/1
  Add2/1 -> Sum/2, Gain5/1
  Constant1/1 -> Sum/1
  NOT/1 -> q-axis current PI/2, Gain2/1
  Gain2/1 -> d-axis current PI/2
  Relay/1 -> NOT/1, Con/1

== system VSCHVDCunitblackstart/Control/Sending-end and receiving-end control/Offshore Control/Control/DC voltage and reactive power control ==
  VdcRef : Inport
  Vdcp : Inport  Port=2
  Vdcn : Inport  Port=3
  Qref : Inport  Port=4
  Qmea : Inport  Port=5
  Con : Inport  Port=6
  Add2 : Sum
  Gain : Gain  Gain=-1
  Gain1 : Gain  Gain=VdcRated/Vbase
  Gain2 : Gain  Gain=0.5
  P PI : slpidlib/PID Controller  Controller=PI  Form=Parallel  TimeDomain=Discrete-time  UseExternalTs=off  SampleTime=Tsc  IntegratorMethod=Forward Euler  FilterMethod=Forward Euler  ControllerParametersSource=internal  P=REnd_Vdc_PI(1)  I=REnd_Vdc_PI(2)  UseKiTs=off  D=0  UseExternalDerivativeSource=off  N=100  UseFilter=on  TunerSelectOption=Transfer Function Based (PID Tuner App)  InitialConditionSource=internal  InitialConditionForIntegrator=0  InitialConditionForFilter=0  DifferentiatorICPrevScaledInput=0  ExternalReset=rising  IgnoreLimit=on  TrackingMode=off  Kt=1  LimitOutput=on  SatLimitsSource=internal  UpperSaturationLimit=1.5  LowerSaturationLimit=-1.5  LinearizeAsGain=on  AntiWindupMode=back-calculation  Kb=1000  LimitIntegrator=off  UpperIntegratorSaturationLimit=inf  LowerIntegratorSaturationLimit=-inf  POutMin=[]  POutMax=[]  IOutMin=[]  IOutMax=[]  DOutMin=[]  DOutMax=[]  NOutMin=[]  NOutMax=[]  SumOutMin=[]  SumOutMax=[]  SaturationOutMin=[]  SaturationOutMax=[]  PParamMin=[]  PParamMax=[]  IParamMin=[]  IParamMax=[]  DParamMin=[]  DParamMax=[]  NParamMin=[]  NParamMax=[]  KbParamMin=[]  KbParamMax=[]  KtParamMin=[]  KtParamMax=[]  KbOutMin=[]  KbOutMax=[]  KtOutMin=[]  KtOutMax=[]  IntegratorOutMin=[]  IntegratorOutMax=[]  FilterOutMin=[]  FilterOutMax=[]  SumI1OutMin=[]  SumI1OutMax=[]  SumI2OutMin=[]  SumI2OutMax=[]  SumI3OutMin=[]  SumI3OutMax=[]  SumI4OutMin=[]  SumI4OutMax=[]  SumDOutMin=[]  SumDOutMax=[]  DifferentiatorOutMin=[]  DifferentiatorOutMax=[]  FilterDiffOutCoefMin=[]  FilterDiffOutCoefMax=[]  ReciprocalOutMin=[]  ReciprocalOutMax=[]  SumDenOutMin=[]  SumDenOutMax=[]  SumNumOutMin=[]  SumNumOutMax=[]  DivideOutMin=[]  DivideOutMax=[]  UdiffTsProdOutMin=[]  UdiffTsProdOutMax=[]  NTsProdOutMin=[]  NTsProdOutMax=[]  UintegralTsProdOutMin=[]  UintegralTsProdOutMax=[]  UngainTsProdOutMin=[]  UngainTsProdOutMax=[]  ClampingZeroOutDataTypeStr=Inherit: Inherit via back propagation  ClampingZeroOutMin=[]  ClampingZeroOutMax=[]  FilterDenConstantOutDataTypeStr=Inherit: Inherit via back propagation  FilterDenConstantOutMin=[]  FilterDenConstantOutMax=[]  PCopyOutDataTypeStr=Inherit: Inherit via back propagation  PCopyOutMin=[]  PCopyOutMax=[]  NCopyOutDataTypeStr=Inherit: Inherit via back propagation  NCopyOutMin=[]  NCopyOutMax=[]  IntegratorContinuousStateAttributes=''  IntegratorStateMustResolveToSignalObject=off  IntegratorRTWStateStorageClass=Auto  FilterContinuousStateAttributes=''  FilterStateMustResolveToSignalObject=off  FilterRTWStateStorageClass=Auto  ParallelPVariant=InternalParameters  IdealPVariant=Disabled  IVariant=InternalParameters  DVariant=Disabled  IntegratorVariant=Discrete  SatVariant=Enabled  AWVariant=BackCalculation  PCopyVariant=Disabled  TRVariant=Disabled  FdbkBlocksVariant=Forward  IdealPFdbkVariant=Disabled  SatFdbkVariant=Disabled  DerivativeFilterVariant=Disabled  NVariant=Disabled  NCopyVariant=Disabled_SignalSpec  FilterICVariant=Disabled  IntegratorICVariant=InternalICs  ExternalResetVariant=ExternalReset  TRSumVariant=Passthrough  SumFdbkVariant=Disabled  SumVariant=Sum_PI  TsampFilterVariant=InternalTs  TsampNgainVariant=Passthrough  TsampIntegralVariant=Disabled_SignalSpec  ExternalSaturationOutDataTypeStr=Inherit: Same as second input  DerivativeSourceVariant=Disabled  PreIntVariant=InternalPreInt
  Q PI : slpidlib/PID Controller  Controller=PI  Form=Parallel  TimeDomain=Discrete-time  UseExternalTs=off  SampleTime=Tsc  IntegratorMethod=Forward Euler  FilterMethod=Forward Euler  ControllerParametersSource=internal  P=REnd_Q_PI(1)  I=REnd_Q_PI(2)  UseKiTs=off  D=0  UseExternalDerivativeSource=off  N=100  UseFilter=on  TunerSelectOption=Transfer Function Based (PID Tuner App)  InitialConditionSource=internal  InitialConditionForIntegrator=0  InitialConditionForFilter=0  DifferentiatorICPrevScaledInput=0  ExternalReset=rising  TrackingMode=off  Kt=1  LimitOutput=on  SatLimitsSource=internal  UpperSaturationLimit=1.5  LowerSaturationLimit=-1.5  LinearizeAsGain=on  AntiWindupMode=back-calculation  Kb=1000  LimitIntegrator=off  UpperIntegratorSaturationLimit=inf  LowerIntegratorSaturationLimit=-inf  POutMin=[]  POutMax=[]  IOutMin=[]  IOutMax=[]  DOutMin=[]  DOutMax=[]  NOutMin=[]  NOutMax=[]  SumOutMin=[]  SumOutMax=[]  SaturationOutMin=[]  SaturationOutMax=[]  PParamMin=[]  PParamMax=[]  IParamMin=[]  IParamMax=[]  DParamMin=[]  DParamMax=[]  NParamMin=[]  NParamMax=[]  KbParamMin=[]  KbParamMax=[]  KtParamMin=[]  KtParamMax=[]  KbOutMin=[]  KbOutMax=[]  KtOutMin=[]  KtOutMax=[]  IntegratorOutMin=[]  IntegratorOutMax=[]  FilterOutMin=[]  FilterOutMax=[]  SumI1OutMin=[]  SumI1OutMax=[]  SumI2OutMin=[]  SumI2OutMax=[]  SumI3OutMin=[]  SumI3OutMax=[]  SumI4OutMin=[]  SumI4OutMax=[]  SumDOutMin=[]  SumDOutMax=[]  DifferentiatorOutMin=[]  DifferentiatorOutMax=[]  FilterDiffOutCoefMin=[]  FilterDiffOutCoefMax=[]  ReciprocalOutMin=[]  ReciprocalOutMax=[]  SumDenOutMin=[]  SumDenOutMax=[]  SumNumOutMin=[]  SumNumOutMax=[]  DivideOutMin=[]  DivideOutMax=[]  UdiffTsProdOutMin=[]  UdiffTsProdOutMax=[]  NTsProdOutMin=[]  NTsProdOutMax=[]  UintegralTsProdOutMin=[]  UintegralTsProdOutMax=[]  UngainTsProdOutMin=[]  UngainTsProdOutMax=[]  ClampingZeroOutDataTypeStr=Inherit: Inherit via back propagation  ClampingZeroOutMin=[]  ClampingZeroOutMax=[]  FilterDenConstantOutDataTypeStr=Inherit: Inherit via back propagation  FilterDenConstantOutMin=[]  FilterDenConstantOutMax=[]  PCopyOutDataTypeStr=Inherit: Inherit via back propagation  PCopyOutMin=[]  PCopyOutMax=[]  NCopyOutDataTypeStr=Inherit: Inherit via back propagation  NCopyOutMin=[]  NCopyOutMax=[]  IntegratorContinuousStateAttributes=''  IntegratorStateMustResolveToSignalObject=off  IntegratorRTWStateStorageClass=Auto  FilterContinuousStateAttributes=''  FilterStateMustResolveToSignalObject=off  FilterRTWStateStorageClass=Auto  ParallelPVariant=InternalParameters  IdealPVariant=Disabled  IVariant=InternalParameters  DVariant=Disabled  IntegratorVariant=Discrete  SatVariant=Enabled  AWVariant=BackCalculation  PCopyVariant=Disabled  TRVariant=Disabled  FdbkBlocksVariant=Forward  IdealPFdbkVariant=Disabled  SatFdbkVariant=Disabled  DerivativeFilterVariant=Disabled  NVariant=Disabled  NCopyVariant=Disabled_SignalSpec  FilterICVariant=Disabled  IntegratorICVariant=InternalICs  ExternalResetVariant=ExternalReset  TRSumVariant=Passthrough  SumFdbkVariant=Disabled  SumVariant=Sum_PI  TsampFilterVariant=InternalTs  TsampNgainVariant=Passthrough  TsampIntegralVariant=Disabled_SignalSpec  ExternalSaturationOutDataTypeStr=Inherit: Same as second input  DerivativeSourceVariant=Disabled  PreIntVariant=InternalPreInt
  Sum5 : Sum  Inputs=|+-
  Sum6 : Sum  Inputs=|+-
  idRef : Outport
  iqRef : Outport  Port=2
  wires:
  Sum5/1 -> Gain1/1
  P PI/1 -> idRef/1
  Sum6/1 -> Q PI/1
  Q PI/1 -> Gain/1
  Qref/1 -> Sum6/1
  Qmea/1 -> Sum6/2
  VdcRef/1 -> Sum5/1
  Gain/1 -> iqRef/1
  Add2/1 -> Gain2/1
  Vdcp/1 -> Add2/1
  Vdcn/1 -> Add2/2
  Gain2/1 -> Sum5/2
  Gain1/1 -> P PI/1
  Con/1 -> P PI/2, Q PI/2

== system VSCHVDCunitblackstart/Control/Sending-end and receiving-end control/Offshore Control/Control/PWM generator ==
  Vref : Inport
  Gain4 : Gain  Gain=-1
  Mux2 : Mux  Inputs=2
  Selector : Selector  InputPortWidth=6  IndexOptions=Index vector (dialog)  Indices=[1 4 2 5 3 6]  OutputSizes=1
  S : Outport
  wires:
  Selector/1 -> S/1
  Gain4/1 -> Mux2/1
  Vref/1 -> Gain4/1, Mux2/2
  Mux2/1 -> Selector/1

== system VSCHVDCunitblackstart/Control/Sending-end and receiving-end control/Offshore Control/Measurements/PQ Calculation ==
  Vd : Inport
  Id : Inport  Port=2
  Iq : Inport  Port=3
  Gain : Gain  Gain=-1
  Product : Product
  Product4 : Product
  P : Outport
  Q : Outport  Port=2
  wires:
  Gain/1 -> Q/1
  Product4/1 -> Gain/1
  Iq/1 -> Product4/2
  Id/1 -> Product/2
  Product/1 -> P/1
  Vd/1 -> Product/1, Product4/1

== system VSCHVDCunitblackstart/Control/Sending-end and receiving-end control/Offshore Control/Measurements/Subsystem ==
  In : Inport
  Gain2 : Gain  Gain=2
  Sum2 : Sum  Inputs=+-  InputSameDT=on  SaturateOnIntegerOverflow=on  OutDataTypeStr=Inherit: Same as first input
  Unit Delay4 : UnitDelay  InitialCondition=Iabcgr0  SampleTime=Ts  HasFrameUpgradeWarning=on
  Out : Outport
  wires:
  In/1 -> Unit Delay4/1, Gain2/1
  Gain2/1 -> Sum2/1
  Sum2/1 -> Out/1
  Unit Delay4/1 -> Sum2/2

== system VSCHVDCunitblackstart/Control/Sending-end and receiving-end control/Offshore Control/Measurements/Subsystem1 ==
  In : Inport
  Gain2 : Gain  Gain=2
  Sum2 : Sum  Inputs=+-  InputSameDT=on  SaturateOnIntegerOverflow=on  OutDataTypeStr=Inherit: Same as first input
  Unit Delay4 : UnitDelay  InitialCondition=Vabcgr0  SampleTime=Ts  HasFrameUpgradeWarning=on
  Out : Outport
  wires:
  Unit Delay4/1 -> Sum2/2
  Sum2/1 -> Out/1
  Gain2/1 -> Sum2/1
  In/1 -> Gain2/1, Unit Delay4/1
